simulink model "sim3"  (R2024a)
settings: Solver=FixedStepAuto  StartTime=0.0  StopTime=10.0  FixedStep=0.55  RelTol=1e-3
libraries: simulink x1
settings Model: Creator=alexe  LastModifiedBy=alexe

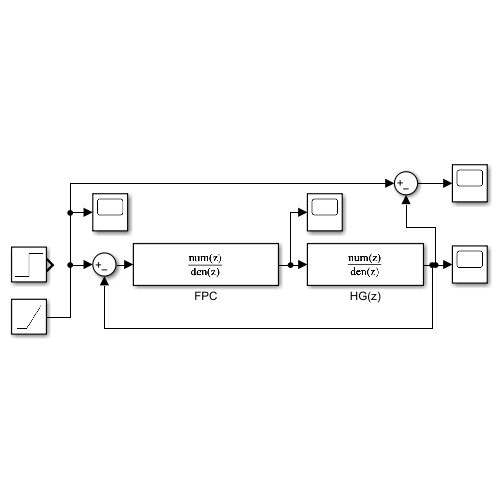
[thumbnail: Simulink's stored preview of the top-level diagram]
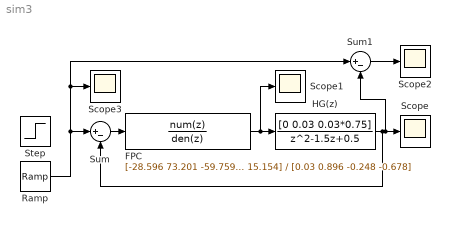
== system sim3 ==
  FPC : DiscreteTransferFcn  Numerator=[-28.596 73.201 -59.759 15.154]  Denominator=[0.03 0.896 -0.248 -0.678]
  HG(z) : DiscreteTransferFcn  Numerator=[0 0.03 0.03*0.75]  Denominator=[1 -1.5 0.5]
  Ramp : simulink/Sources/Ramp  slope=1  start=0  InitialOutput=1
  Scope{,1..3} (4 alike) : Scope
  Step : Step  Before=1
  Sum : Sum  Inputs=|+-
  Sum1 : Sum  Inputs=|+-
  wires:
  Sum/1 -> FPC/1
  FPC/1 -> Scope1/1, HG(z)/1
  HG(z)/1 -> Sum/2, Sum1/2, Scope/1
  Sum1/1 -> Scope2/1
  Ramp/1 -> Sum/1, Scope3/1, Sum1/1
